simulink model "Torque_controller_IFOC"  (R2023b)
settings: Solver=ode5  StartTime=0.0  StopTime=tsim  FixedStep=tstep  MaxStep=1e-4  RelTol=1e-3
undefined symbols (not defined in the file or in its folder): MI_Contr, MI_contr, MI_motor, tau_L, tau_Rref
libraries: simulink x6, mcbcontrolslib x2, spsRMSLib x2
settings Model: Creator=HP  LastModifiedBy=HP

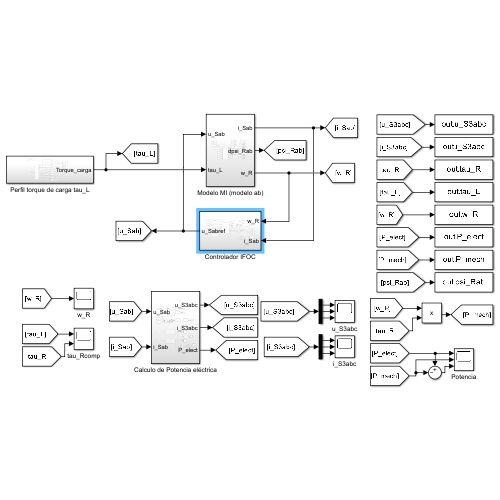
[thumbnail: Simulink's stored preview of the top-level diagram]
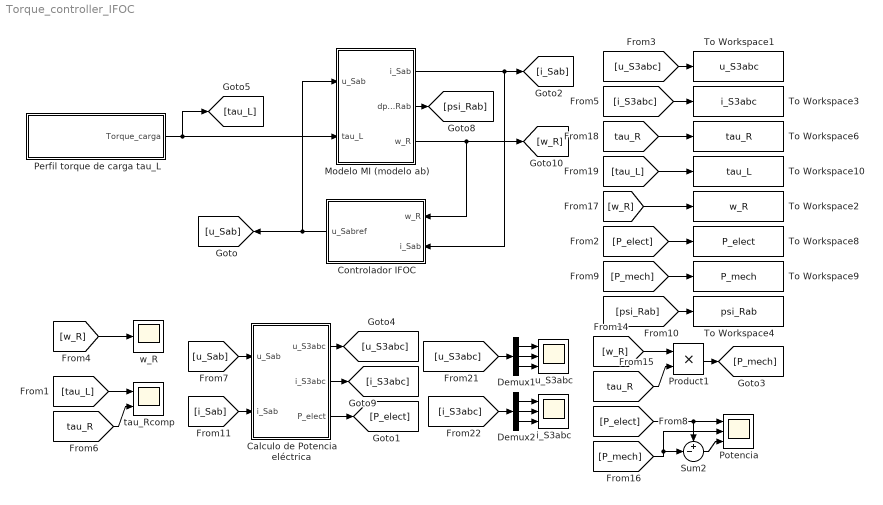
== system Torque_controller_IFOC ==
  Calculo de Potencia eléctrica : Subsystem
  Controlador IFOC : Subsystem
  Demux1 : Demux  Outputs=3
  Demux2 : Demux  Outputs=3
  Modelo MI (modelo ab) : Subsystem
  Perfil torque de carga tau_L : Subsystem
  Potencia : Scope  NumInputPorts=3
  Product1 : Product
  Sum2 : Sum  Inputs=+-|
  To Workspace1 : ToWorkspace  VariableName=u_S3abc  SaveFormat=Timeseries  SampleTime=-1
  To Workspace10 : ToWorkspace  VariableName=tau_L  SaveFormat=Timeseries  SampleTime=-1
  To Workspace2 : ToWorkspace  VariableName=w_R  SaveFormat=Timeseries  SampleTime=-1
  To Workspace3 : ToWorkspace  VariableName=i_S3abc  SaveFormat=Timeseries  SampleTime=-1
  To Workspace4 : ToWorkspace  VariableName=psi_Rab  SaveFormat=Timeseries  SampleTime=-1
  To Workspace6 : ToWorkspace  VariableName=tau_R  SaveFormat=Timeseries  SampleTime=-1
  To Workspace8 : ToWorkspace  VariableName=P_elect  SaveFormat=Timeseries  SampleTime=-1
  To Workspace9 : ToWorkspace  VariableName=P_mech  SaveFormat=Timeseries  SampleTime=-1
  i_S3abc : Scope  NumInputPorts=3
  tau_Rcomp : Scope  NumInputPorts=2
  u_S3abc : Scope  NumInputPorts=3
  w_R : Scope
  wires:
  Modelo MI (modelo ab)/1(i_Sab) -> [i_Sab], Controlador IFOC/2(i_Sab)
  Modelo MI (modelo ab)/3(w_R) -> Controlador IFOC/1(w_R), [w_R]
  Controlador IFOC/1(u_Sabref) -> Modelo MI (modelo ab)/1(u_Sab), [u_Sab]
  Modelo MI (modelo ab)/2(dpsi_Rab) -> [psi_Rab]
  Perfil torque de carga tau_L/1(Torque_carga) -> Modelo MI (modelo ab)/2(tau_L), [tau_L]
  Calculo de Potencia eléctrica/1(u_S3abc) -> [u_S3abc]
  Calculo de Potencia eléctrica/3(P_elect) -> [P_elect]
  Product1/1 -> [P_mech]
  [i_S3abc] -> Demux2/1
  [w_R] -> Product1/1
  [tau_R] -> Product1/2
  [P_elect] -> Potencia/1, Sum2/1
  [u_S3abc] -> Demux1/1
  Demux1/1 -> u_S3abc/1
  [i_Sab] -> Calculo de Potencia eléctrica/2(i_Sab)
  Calculo de Potencia eléctrica/2(i_S3abc) -> [i_S3abc]
  Sum2/1 -> Potencia/3
  Demux1/3 -> u_S3abc/3
  [P_mech] -> Potencia/2, Sum2/2
  Demux2/1 -> i_S3abc/1
  [tau_L] -> tau_Rcomp/1
  [tau_R] -> tau_Rcomp/2
  Demux2/2 -> i_S3abc/2
  Demux2/3 -> i_S3abc/3
  Demux1/2 -> u_S3abc/2
  [u_Sab] -> Calculo de Potencia eléctrica/1(u_Sab)
  [P_elect] -> To Workspace8/1
  [w_R] -> To Workspace2/1
  [i_S3abc] -> To Workspace3/1
  [psi_Rab] -> To Workspace4/1
  [tau_L] -> To Workspace10/1
  [P_mech] -> To Workspace9/1
  [tau_R] -> To Workspace6/1
  [u_S3abc] -> To Workspace1/1
  [w_R] -> w_R/1

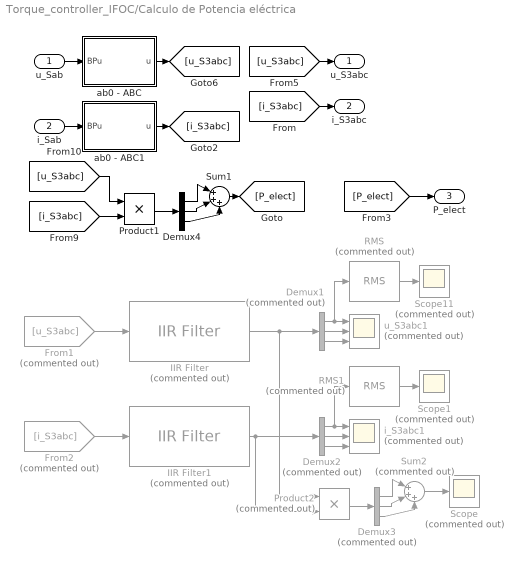
== system Torque_controller_IFOC/Calculo de Potencia eléctrica ==
  u_Sab : Inport
  i_Sab : Inport  Port=2
  Demux1 : Demux  Commented=on  Outputs=3
  Demux2 : Demux  Commented=on  Outputs=3
  Demux3 : Demux  Commented=on  Outputs=3
  Demux4 : Demux  Outputs=3
  From1 : From  Commented=on  GotoTag=u_S3abc
  From2 : From  Commented=on  GotoTag=i_S3abc
  IIR Filter : mcbcontrolslib/IIR Filter  Commented=on  VariantControl=Low Pass Filter  VariantSelect=Low-pass  Filter_constant=0.04  advancedSettings=on  Ts=50e-6  cutOff_freq=132.6291
      settings: LibrarySourceBlock=mcbhdllib/Signal Management/IIR Filter
  IIR Filter1 : mcbcontrolslib/IIR Filter  Commented=on  VariantControl=Low Pass Filter  VariantSelect=Low-pass  Filter_constant=0.04  advancedSettings=on  Ts=50e-6  cutOff_freq=132.6291
      settings: LibrarySourceBlock=mcbhdllib/Signal Management/IIR Filter
  Product1 : Product
  Product2 : Product  Commented=on
  RMS : spsRMSLib/RMS  Commented=on  TrueRMS=on  Freq=60  RMSInit=120  Ts=0
  RMS1 : spsRMSLib/RMS  Commented=on  TrueRMS=on  Freq=60  RMSInit=120  Ts=0
  Scope : Scope  Commented=on
  Scope1 : Scope  Commented=on
  Scope11 : Scope  Commented=on
  Sum1 : Sum  Inputs=|+++
  Sum2 : Sum  Commented=on  Inputs=|+++
  ab0 - ABC : MATLAB Function  TreatAsAtomicUnit=on
  ab0 - ABC1 : MATLAB Function  TreatAsAtomicUnit=on
  i_S3abc1 : Scope  Commented=on  NumInputPorts=3
  u_S3abc1 : Scope  Commented=on  NumInputPorts=3
  u_S3abc : Outport
  i_S3abc : Outport  Port=2
  P_elect : Outport  Port=3
  wires:
  Demux4/1 -> Sum1/1
  [i_S3abc] -> Product1/2
  i_Sab/1 -> ab0 - ABC1/1(BPu)
  Demux4/3 -> Sum1/3
  [u_S3abc] -> Product1/1
  Demux4/2 -> Sum1/2
  Product1/1 -> Demux4/1
  u_Sab/1 -> ab0 - ABC/1(BPu)
  [u_S3abc] -> u_S3abc/1
  [i_S3abc] -> i_S3abc/1
  ab0 - ABC/1(u) -> [u_S3abc]
  ab0 - ABC1/1(u) -> [i_S3abc]
  IIR Filter/1 -> Product2/1, Demux1/1
  RMS/1 -> Scope11/1
  Demux1/2 -> u_S3abc1/2
  Demux1/3 -> u_S3abc1/3
  Demux1/1 -> RMS/1, u_S3abc1/1
  From1/1 -> IIR Filter/1
  Demux2/1 -> RMS1/1, i_S3abc1/1
  RMS1/1 -> Scope1/1
  Demux2/2 -> i_S3abc1/2
  IIR Filter1/1 -> Product2/2, Demux2/1
  From2/1 -> IIR Filter1/1
  Demux2/3 -> i_S3abc1/3
  Demux3/2 -> Sum2/2
  Demux3/3 -> Sum2/3
  Sum2/1 -> Scope/1
  Product2/1 -> Demux3/1
  Demux3/1 -> Sum2/1
  Sum1/1 -> [P_elect]
  [P_elect] -> P_elect/1

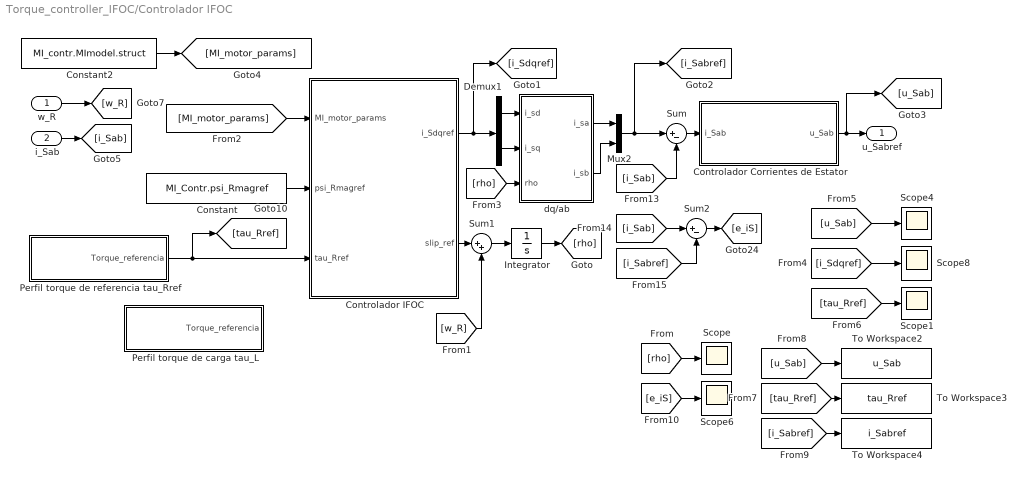
== system Torque_controller_IFOC/Controlador IFOC ==
  w_R : Inport
  i_Sab : Inport  Port=2
  Constant : Constant  Value=MI_Contr.psi_Rmagref
  Constant2 : Constant  Value=MI_contr.MImodel.struct  OutDataTypeStr=Bus: MI_bus
  Controlador Corrientes de Estator : Subsystem
  Controlador IFOC : MATLAB Function  TreatAsAtomicUnit=on
  Demux1 : Demux  Outputs=2
  Integrator : Integrator
  Mux2 : Mux  Inputs=2
  Perfil torque de carga tau_L : Subsystem
  Perfil torque de referencia tau_Rref : Subsystem
  Scope{,1,4,6,8} (5 alike) : Scope
  Sum : Sum  Inputs=|+-
  Sum1 : Sum  Inputs=|++
  Sum2 : Sum  Inputs=|+-
  To Workspace2 : ToWorkspace  VariableName=u_Sab  SaveFormat=Timeseries  SampleTime=-1
  To Workspace3 : ToWorkspace  VariableName=tau_Rref  SaveFormat=Timeseries  SampleTime=-1
  To Workspace4 : ToWorkspace  VariableName=i_Sabref  SaveFormat=Timeseries  SampleTime=-1
  dq/ab : MATLAB Function  TreatAsAtomicUnit=on
  u_Sabref : Outport
  wires:
  Controlador Corrientes de Estator/1(u_Sab) -> [u_Sab], u_Sabref/1
  [i_Sab] -> Sum/2
  Sum/1 -> Controlador Corrientes de Estator/1(i_Sab)
  dq/ab/2(i_sb) -> Mux2/2
  dq/ab/1(i_sa) -> Mux2/1
  Demux1/1 -> dq/ab/1(i_sd)
  Demux1/2 -> dq/ab/2(i_sq)
  Controlador IFOC/1(i_Sdqref) -> [i_Sdqref], Demux1/1
  i_Sab/1 -> [i_Sab]
  Controlador IFOC/2(slip_ref) -> Sum1/1
  w_R/1 -> [w_R]
  [w_R] -> Sum1/2
  Sum1/1 -> Integrator/1
  Integrator/1 -> [rho]
  [MI_motor_params] -> Controlador IFOC/1(MI_motor_params)
  Constant/1 -> Controlador IFOC/2(psi_Rmagref)
  [rho] -> dq/ab/3(rho)
  [i_Sdqref] -> Scope8/1
  [rho] -> Scope/1
  [u_Sab] -> Scope4/1
  [i_Sab] -> Sum2/1
  [i_Sabref] -> Sum2/2
  Mux2/1 -> [i_Sabref], Sum/1
  [tau_Rref] -> Scope1/1
  Perfil torque de referencia tau_Rref/1(Torque_referencia) -> Controlador IFOC/3(tau_Rref), [tau_Rref]
  [u_Sab] -> To Workspace2/1
  [tau_Rref] -> To Workspace3/1
  [i_Sabref] -> To Workspace4/1
  Sum2/1 -> [e_iS]
  [e_iS] -> Scope6/1
  Constant2/1 -> [MI_motor_params]

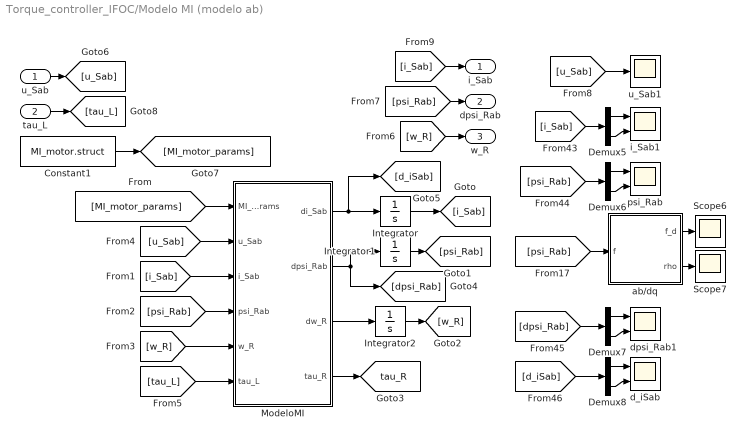
== system Torque_controller_IFOC/Modelo MI (modelo ab) ==
  u_Sab : Inport
  tau_L : Inport  Port=2
  Constant1 : Constant  Value=MI_motor.struct  OutDataTypeStr=Bus: MI_bus
  Demux{5..8} (4 alike) : Demux  Outputs=2
  Integrator : Integrator
  Integrator1 : Integrator
  Integrator2 : Integrator
  ModeloMI : MATLAB Function  TreatAsAtomicUnit=on
  Scope6 : Scope
  Scope7 : Scope
  ab/dq : MATLAB Function  TreatAsAtomicUnit=on
  d_iSab : Scope  NumInputPorts=2
  dpsi_Rab1 : Scope  NumInputPorts=2
  i_Sab1 : Scope  NumInputPorts=2
  psi_Rab : Scope  NumInputPorts=2
  u_Sab1 : Scope
  i_Sab : Outport
  dpsi_Rab : Outport  Port=2
  w_R : Outport  Port=3
  tag scope: tau_R=global
  wires:
  ModeloMI/1(di_Sab) -> Integrator/1, [d_iSab]
  ModeloMI/2(dpsi_Rab) -> [dpsi_Rab], Integrator1/1
  [w_R] -> ModeloMI/5(w_R)
  [psi_Rab] -> ModeloMI/4(psi_Rab)
  Integrator2/1 -> [w_R]
  [i_Sab] -> ModeloMI/3(i_Sab)
  ModeloMI/3(dw_R) -> Integrator2/1
  Integrator1/1 -> [psi_Rab]
  u_Sab/1 -> [u_Sab]
  ModeloMI/4(tau_R) -> [tau_R]
  Demux7/1 -> dpsi_Rab1/1
  Demux7/2 -> dpsi_Rab1/2
  [d_iSab] -> Demux8/1
  Demux8/2 -> d_iSab/2
  Demux8/1 -> d_iSab/1
  [dpsi_Rab] -> Demux7/1
  Integrator/1 -> [i_Sab]
  [MI_motor_params] -> ModeloMI/1(MI_motor_params)
  Constant1/1 -> [MI_motor_params]
  Demux6/2 -> psi_Rab/2
  Demux5/1 -> i_Sab1/1
  [psi_Rab] -> Demux6/1
  Demux5/2 -> i_Sab1/2
  Demux6/1 -> psi_Rab/1
  [u_Sab] -> u_Sab1/1
  [i_Sab] -> Demux5/1
  ab/dq/2(rho) -> Scope7/1
  ab/dq/1(f_d) -> Scope6/1
  [psi_Rab] -> ab/dq/1(f)
  [u_Sab] -> ModeloMI/2(u_Sab)
  tau_L/1 -> [tau_L]
  [tau_L] -> ModeloMI/6(tau_L)
  [i_Sab] -> i_Sab/1
  [psi_Rab] -> dpsi_Rab/1
  [w_R] -> w_R/1

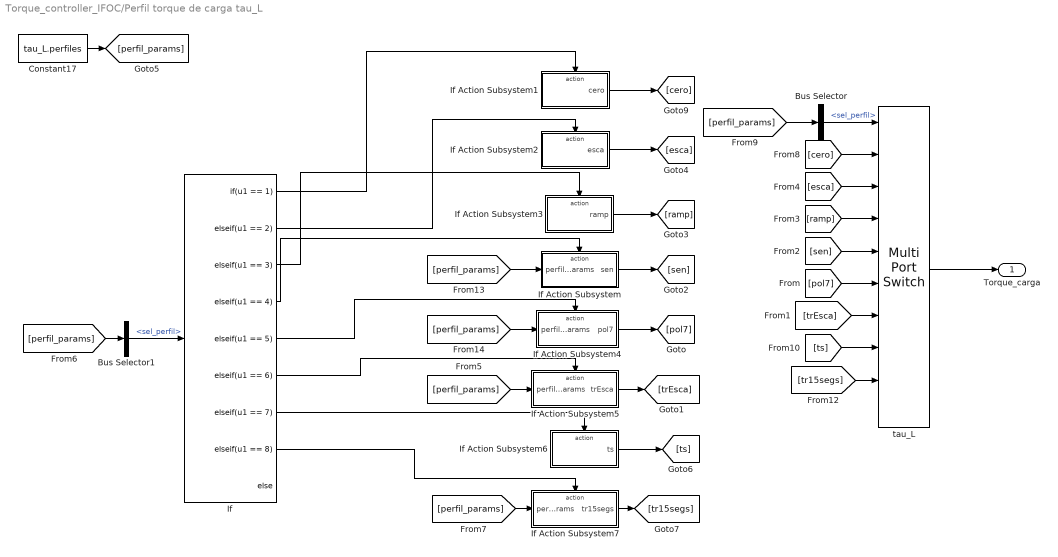
== system Torque_controller_IFOC/Perfil torque de carga tau_L ==
  Bus Selector : BusSelector  OutputSignals=sel_perfil
  Bus Selector1 : BusSelector  OutputSignals=sel_perfil
  Constant17 : Constant  Value=tau_L.perfiles  OutDataTypeStr=Bus: Perfil_bus
  If : If  IfExpression=u1 == 1  ElseIfExpressions=u1 == 2,u1 == 3,u1 == 4,u1 == 5,u1 == 6,u1 == 7,u1 == 8
  If Action Subsystem : Subsystem  TreatAsAtomicUnit=on
  If Action Subsystem1 : Subsystem  TreatAsAtomicUnit=on
  If Action Subsystem2 : Subsystem  TreatAsAtomicUnit=on
  If Action Subsystem3 : Subsystem  TreatAsAtomicUnit=on
  If Action Subsystem4 : Subsystem  TreatAsAtomicUnit=on
  If Action Subsystem5 : Subsystem  TreatAsAtomicUnit=on
  If Action Subsystem6 : Subsystem  TreatAsAtomicUnit=on
  If Action Subsystem7 : Subsystem  TreatAsAtomicUnit=on
  tau_L : MultiPortSwitch  Inputs=9  SaturateOnIntegerOverflow=off  InputSameDT=off
  Torque_carga : Outport
  wires:
  tau_L/1 -> Torque_carga/1
  [ramp] -> tau_L/4
  [trEsca] -> tau_L/7
  [pol7] -> tau_L/6
  [sen] -> tau_L/5
  [esca] -> tau_L/3
  Constant17/1 -> [perfil_params]
  [ts] -> tau_L/8
  [tr15segs] -> tau_L/9
  Bus Selector/1 -> tau_L/1  "<sel_perfil>"
  [perfil_params] -> Bus Selector/1
  If Action Subsystem/1(sen) -> [sen]
  [perfil_params] -> Bus Selector1/1
  Bus Selector1/1 -> If/1  "<sel_perfil>"
  If/4 -> If Action Subsystem/Action
  If Action Subsystem1/1(cero) -> [cero]
  [cero] -> tau_L/2
  [perfil_params] -> If Action Subsystem/1(perfil_params)
  If/1 -> If Action Subsystem1/Action
  If Action Subsystem2/1(esca) -> [esca]
  If/2 -> If Action Subsystem2/Action
  If Action Subsystem3/1(ramp) -> [ramp]
  If/3 -> If Action Subsystem3/Action
  [perfil_params] -> If Action Subsystem4/1(perfil_params)
  If/5 -> If Action Subsystem4/Action
  If Action Subsystem4/1(pol7) -> [pol7]
  If Action Subsystem5/1(trEsca) -> [trEsca]
  [perfil_params] -> If Action Subsystem5/1(perfil_params)
  If Action Subsystem6/1(ts) -> [ts]
  If/6 -> If Action Subsystem5/Action
  If/7 -> If Action Subsystem6/Action
  If Action Subsystem7/1(tr15segs) -> [tr15segs]
  If/8 -> If Action Subsystem7/Action
  [perfil_params] -> If Action Subsystem7/1(perfil_params)

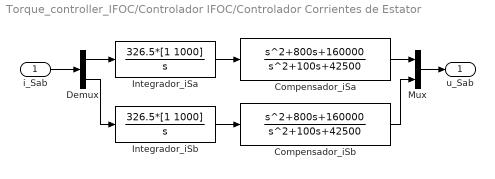
== system Torque_controller_IFOC/Controlador IFOC/Controlador Corrientes de Estator ==
  i_Sab : Inport
  Compensador_iSa : TransferFcn  Numerator=[1,800,160000]  Denominator=[1,100,42500]
  Compensador_iSb : TransferFcn  Numerator=[1,800,160000]  Denominator=[1,100,42500]
  Demux : Demux  Outputs=2
  Integrador_iSa : TransferFcn  Numerator=326.5*[1 1000]  Denominator=[1 0]
  Integrador_iSb : TransferFcn  Numerator=326.5*[1 1000]  Denominator=[1 0]
  Mux : Mux  Inputs=2
  u_Sab : Outport
  wires:
  Integrador_iSa/1 -> Compensador_iSa/1
  Integrador_iSb/1 -> Compensador_iSb/1
  i_Sab/1 -> Demux/1
  Demux/1 -> Integrador_iSa/1
  Demux/2 -> Integrador_iSb/1
  Compensador_iSa/1 -> Mux/1
  Mux/1 -> u_Sab/1
  Compensador_iSb/1 -> Mux/2

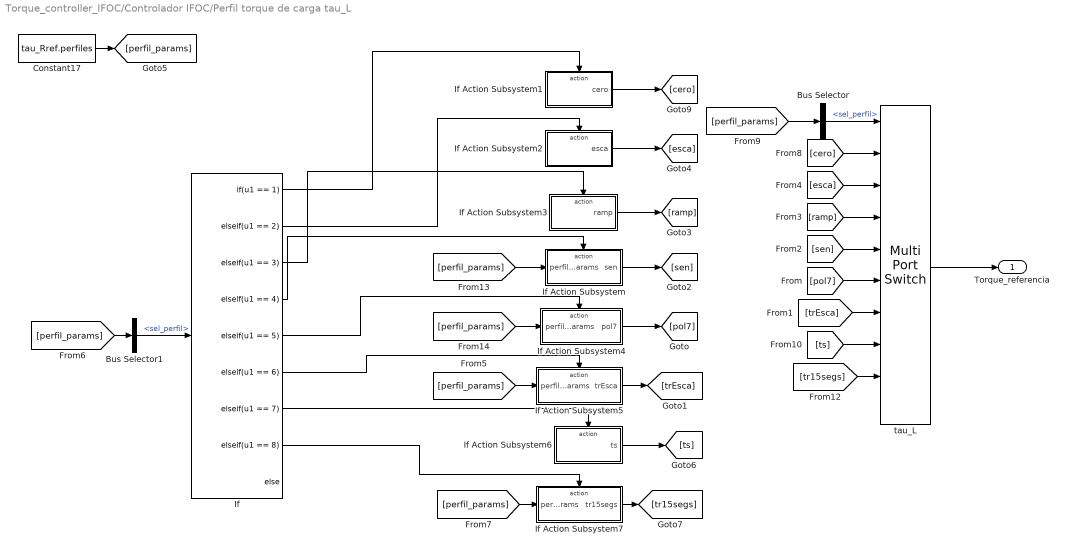
== system Torque_controller_IFOC/Controlador IFOC/Perfil torque de carga tau_L ==
  Bus Selector : BusSelector  OutputSignals=sel_perfil
  Bus Selector1 : BusSelector  OutputSignals=sel_perfil
  Constant17 : Constant  Value=tau_Rref.perfiles  OutDataTypeStr=Bus: Perfil_bus
  If : If  IfExpression=u1 == 1  ElseIfExpressions=u1 == 2,u1 == 3,u1 == 4,u1 == 5,u1 == 6,u1 == 7,u1 == 8
  If Action Subsystem : Subsystem  TreatAsAtomicUnit=on
  If Action Subsystem1 : Subsystem  TreatAsAtomicUnit=on
  If Action Subsystem2 : Subsystem  TreatAsAtomicUnit=on
  If Action Subsystem3 : Subsystem  TreatAsAtomicUnit=on
  If Action Subsystem4 : Subsystem  TreatAsAtomicUnit=on
  If Action Subsystem5 : Subsystem  TreatAsAtomicUnit=on
  If Action Subsystem6 : Subsystem  TreatAsAtomicUnit=on
  If Action Subsystem7 : Subsystem  TreatAsAtomicUnit=on
  tau_L : MultiPortSwitch  Inputs=9  SaturateOnIntegerOverflow=off  InputSameDT=off
  Torque_referencia : Outport
  wires:
  tau_L/1 -> Torque_referencia/1
  [ramp] -> tau_L/4
  [trEsca] -> tau_L/7
  [pol7] -> tau_L/6
  [sen] -> tau_L/5
  [esca] -> tau_L/3
  Constant17/1 -> [perfil_params]
  [ts] -> tau_L/8
  [tr15segs] -> tau_L/9
  Bus Selector/1 -> tau_L/1  "<sel_perfil>"
  [perfil_params] -> Bus Selector/1
  If Action Subsystem/1(sen) -> [sen]
  [perfil_params] -> Bus Selector1/1
  Bus Selector1/1 -> If/1  "<sel_perfil>"
  If/4 -> If Action Subsystem/Action
  If Action Subsystem1/1(cero) -> [cero]
  [cero] -> tau_L/2
  [perfil_params] -> If Action Subsystem/1(perfil_params)
  If/1 -> If Action Subsystem1/Action
  If Action Subsystem2/1(esca) -> [esca]
  If/2 -> If Action Subsystem2/Action
  If Action Subsystem3/1(ramp) -> [ramp]
  If/3 -> If Action Subsystem3/Action
  [perfil_params] -> If Action Subsystem4/1(perfil_params)
  If/5 -> If Action Subsystem4/Action
  If Action Subsystem4/1(pol7) -> [pol7]
  If Action Subsystem5/1(trEsca) -> [trEsca]
  [perfil_params] -> If Action Subsystem5/1(perfil_params)
  If Action Subsystem6/1(ts) -> [ts]
  If/6 -> If Action Subsystem5/Action
  If/7 -> If Action Subsystem6/Action
  If Action Subsystem7/1(tr15segs) -> [tr15segs]
  If/8 -> If Action Subsystem7/Action
  [perfil_params] -> If Action Subsystem7/1(perfil_params)

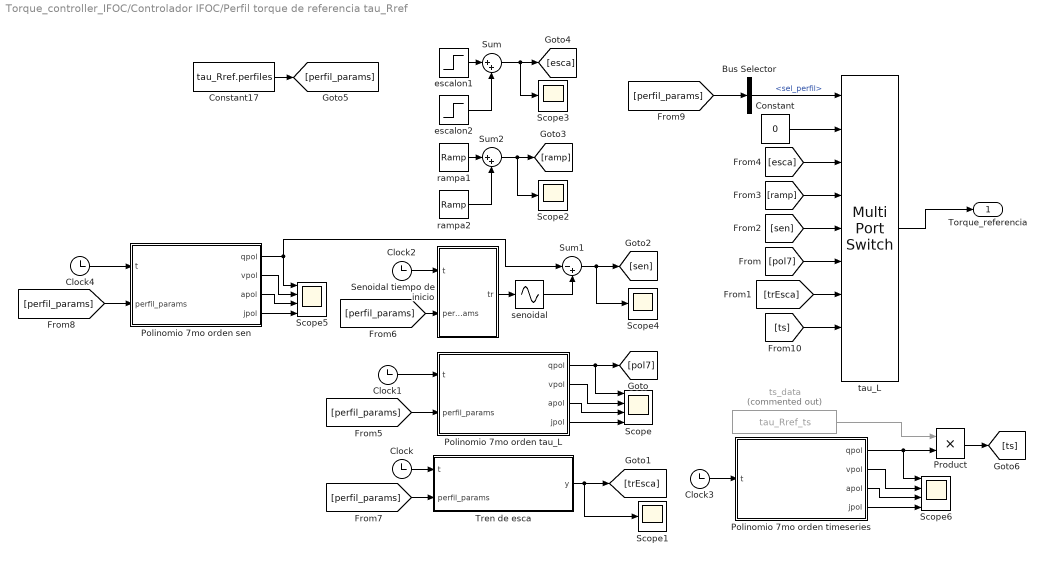
== system Torque_controller_IFOC/Controlador IFOC/Perfil torque de referencia tau_Rref ==
  Bus Selector : BusSelector  OutputSignals=sel_perfil
  Clock{,1..4} (5 alike) : Clock
  Constant : Constant  Value=0
  Constant17 : Constant  Value=tau_Rref.perfiles  OutDataTypeStr=Bus: Perfil_bus
  Polinomio 7mo orden sen : MATLAB Function  TreatAsAtomicUnit=on
  Polinomio 7mo orden tau_L : MATLAB Function  TreatAsAtomicUnit=on
  Polinomio 7mo orden timeseries : MATLAB Function  TreatAsAtomicUnit=on
  Product : Product
  Scope : Scope  NumInputPorts=4
  Scope{1..4} (4 alike) : Scope
  Scope5 : Scope  NumInputPorts=4
  Scope6 : Scope  NumInputPorts=4
  Senoidal tiempo de inicio : MATLAB Function  TreatAsAtomicUnit=on
  Sum : Sum  Inputs=|++
  Sum1 : Sum  Inputs=|-+
  Sum2 : Sum  Inputs=|++
  Tren de esca : MATLAB Function  TreatAsAtomicUnit=on
  escalon1 : Step  Time=2.5  After=0.85  SampleTime=0
  escalon2 : Step  Time=7.5  After=-0.85  SampleTime=0
  rampa1 : simulink/Sources/Ramp  slope=0.02064  start=2.5  InitialOutput=0
  rampa2 : simulink/Sources/Ramp  slope=-0.02064  start=7.5  InitialOutput=0
  senoidal : Sin  TimeSource=Use external signal  Amplitude=0.41519  Frequency=6.2832  Phase=1.5708  SampleTime=0
  tau_L : MultiPortSwitch  Inputs=8  SaturateOnIntegerOverflow=off  InputSameDT=off
  ts_data : FromWorkspace  Commented=on  VariableName=tau_Rref_ts
  Torque_referencia : Outport
  wires:
  Polinomio 7mo orden tau_L/2(vpol) -> Scope/2
  Polinomio 7mo orden tau_L/3(apol) -> Scope/3
  Polinomio 7mo orden tau_L/4(jpol) -> Scope/4
  Sum2/1 -> Scope2/1, [ramp]
  Constant/1 -> tau_L/2
  rampa2/1 -> Sum2/2
  rampa1/1 -> Sum2/1
  tau_L/1 -> Torque_referencia/1
  Clock/1 -> Tren de esca/1(t)
  Tren de esca/1(y) -> Scope1/1, [trEsca]
  Polinomio 7mo orden tau_L/1(qpol) -> Scope/1, [pol7]
  escalon1/1 -> Sum/1
  Sum/1 -> [esca], Scope3/1
  escalon2/1 -> Sum/2
  [ramp] -> tau_L/4
  [trEsca] -> tau_L/7
  [pol7] -> tau_L/6
  [sen] -> tau_L/5
  [esca] -> tau_L/3
  Clock2/1 -> Senoidal tiempo de inicio/1(t)
  Senoidal tiempo de inicio/1(tr) -> senoidal/1
  Constant17/1 -> [perfil_params]
  Clock1/1 -> Polinomio 7mo orden tau_L/1(t)
  [perfil_params] -> Polinomio 7mo orden tau_L/2(perfil_params)
  [perfil_params] -> Senoidal tiempo de inicio/2(perfil_params)
  [perfil_params] -> Tren de esca/2(perfil_params)
  Clock4/1 -> Polinomio 7mo orden sen/1(t)
  [perfil_params] -> Polinomio 7mo orden sen/2(perfil_params)
  senoidal/1 -> Sum1/2
  Polinomio 7mo orden sen/2(vpol) -> Scope5/2
  Polinomio 7mo orden sen/3(apol) -> Scope5/3
  Polinomio 7mo orden sen/4(jpol) -> Scope5/4
  Polinomio 7mo orden sen/1(qpol) -> Sum1/1, Scope5/1
  Sum1/1 -> Scope4/1, [sen]
  Bus Selector/1 -> tau_L/1  "<sel_perfil>"
  [perfil_params] -> Bus Selector/1
  Clock3/1 -> Polinomio 7mo orden timeseries/1(t)
  Polinomio 7mo orden timeseries/2(vpol) -> Scope6/2
  Polinomio 7mo orden timeseries/1(qpol) -> Product/2, Scope6/1
  Polinomio 7mo orden timeseries/4(jpol) -> Scope6/4
  Polinomio 7mo orden timeseries/3(apol) -> Scope6/3
  ts_data/1 -> Product/1
  Product/1 -> [ts]
  [ts] -> tau_L/8

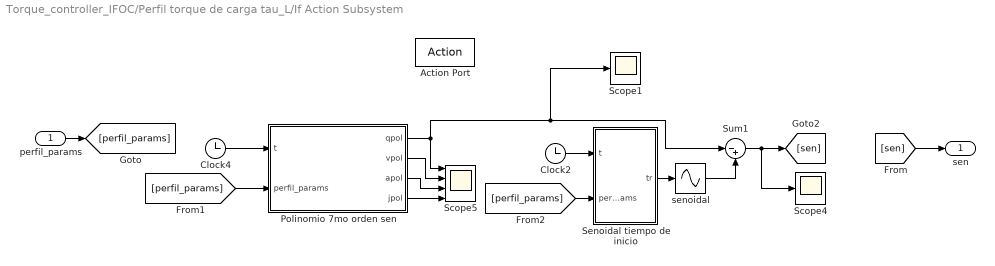
== system Torque_controller_IFOC/Perfil torque de carga tau_L/If Action Subsystem ==
  perfil_params : Inport
  Action Port : ActionPort
  Clock2 : Clock
  Clock4 : Clock
  Polinomio 7mo orden sen : MATLAB Function  TreatAsAtomicUnit=on
  Scope1 : Scope
  Scope4 : Scope
  Scope5 : Scope  NumInputPorts=4
  Senoidal tiempo de inicio : MATLAB Function  TreatAsAtomicUnit=on
  Sum1 : Sum  Inputs=|-+
  senoidal : Sin  TimeSource=Use external signal  Frequency=6.2832  Phase=1.5708  SampleTime=0
  sen : Outport
  wires:
  Clock4/1 -> Polinomio 7mo orden sen/1(t)
  Polinomio 7mo orden sen/1(qpol) -> Scope1/1, Sum1/1, Scope5/1
  Sum1/1 -> Scope4/1, [sen]
  Polinomio 7mo orden sen/4(jpol) -> Scope5/4
  Polinomio 7mo orden sen/3(apol) -> Scope5/3
  Clock2/1 -> Senoidal tiempo de inicio/1(t)
  [perfil_params] -> Polinomio 7mo orden sen/2(perfil_params)
  Polinomio 7mo orden sen/2(vpol) -> Scope5/2
  senoidal/1 -> Sum1/2
  Senoidal tiempo de inicio/1(tr) -> senoidal/1
  [sen] -> sen/1
  perfil_params/1 -> [perfil_params]
  [perfil_params] -> Senoidal tiempo de inicio/2(perfil_params)

== system Torque_controller_IFOC/Perfil torque de carga tau_L/If Action Subsystem1 ==
  Action Port : ActionPort
  Constant : Constant  Value=0
  cero : Outport
  wires:
  Constant/1 -> cero/1

== system Torque_controller_IFOC/Perfil torque de carga tau_L/If Action Subsystem2 ==
  Action Port : ActionPort
  Scope3 : Scope
  Sum : Sum  Inputs=|++
  escalon1 : Step  Time=2.5  After=0.70582  SampleTime=0
  escalon2 : Step  Time=7.5  After=-0.70582  SampleTime=0
  esca : Outport
  wires:
  escalon2/1 -> Sum/2
  escalon1/1 -> Sum/1
  Sum/1 -> [esca], Scope3/1
  [esca] -> esca/1

== system Torque_controller_IFOC/Perfil torque de carga tau_L/If Action Subsystem3 ==
  Action Port : ActionPort
  Scope2 : Scope
  Sum2 : Sum  Inputs=|++
  rampa1 : simulink/Sources/Ramp  slope=0.02064  start=2.5  InitialOutput=0
  rampa2 : simulink/Sources/Ramp  slope=-0.02064  start=7.5  InitialOutput=0
  ramp : Outport
  wires:
  rampa2/1 -> Sum2/2
  rampa1/1 -> Sum2/1
  Sum2/1 -> Scope2/1, [ramp]
  [ramp] -> ramp/1

== system Torque_controller_IFOC/Perfil torque de carga tau_L/If Action Subsystem4 ==
  perfil_params : Inport
  Action Port : ActionPort
  Clock1 : Clock
  Polinomio 7mo orden tau_L : MATLAB Function  TreatAsAtomicUnit=on
  Scope : Scope  NumInputPorts=4
  pol7 : Outport
  wires:
  Polinomio 7mo orden tau_L/4(jpol) -> Scope/4
  Polinomio 7mo orden tau_L/1(qpol) -> Scope/1, [pol7]
  Polinomio 7mo orden tau_L/2(vpol) -> Scope/2
  Clock1/1 -> Polinomio 7mo orden tau_L/1(t)
  Polinomio 7mo orden tau_L/3(apol) -> Scope/3
  perfil_params/1 -> Polinomio 7mo orden tau_L/2(perfil_params)
  [pol7] -> pol7/1

== system Torque_controller_IFOC/Perfil torque de carga tau_L/If Action Subsystem5 ==
  perfil_params : Inport
  Action Port : ActionPort
  Clock : Clock
  Scope1 : Scope
  Tren de esca : MATLAB Function  TreatAsAtomicUnit=on
  trEsca : Outport
  wires:
  Tren de esca/1(q) -> Scope1/1, [trEsca]
  Clock/1 -> Tren de esca/1(t)
  perfil_params/1 -> Tren de esca/2(perfil_params)
  [trEsca] -> trEsca/1

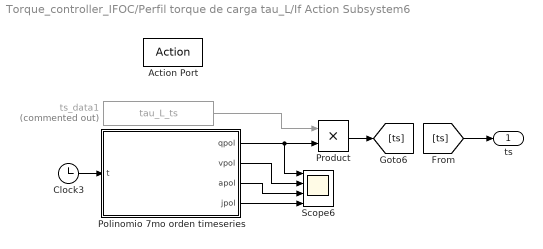
== system Torque_controller_IFOC/Perfil torque de carga tau_L/If Action Subsystem6 ==
  Action Port : ActionPort
  Clock3 : Clock
  Polinomio 7mo orden timeseries : MATLAB Function  TreatAsAtomicUnit=on
  Product : Product
  Scope6 : Scope  NumInputPorts=4
  ts_data1 : FromWorkspace  Commented=on  VariableName=tau_L_ts
  ts : Outport
  wires:
  Product/1 -> [ts]
  Clock3/1 -> Polinomio 7mo orden timeseries/1(t)
  ts_data1/1 -> Product/1
  Polinomio 7mo orden timeseries/4(jpol) -> Scope6/4
  Polinomio 7mo orden timeseries/2(vpol) -> Scope6/2
  Polinomio 7mo orden timeseries/3(apol) -> Scope6/3
  Polinomio 7mo orden timeseries/1(qpol) -> Product/2, Scope6/1
  [ts] -> ts/1

== system Torque_controller_IFOC/Perfil torque de carga tau_L/If Action Subsystem7 ==
  perfil_params : Inport
  Action Port : ActionPort
  Clock5 : Clock
  Scope7 : Scope
  Trayectoria 15 segmentos : MATLAB Function  TreatAsAtomicUnit=on
  tr15segs : Outport
  wires:
  Clock5/1 -> Trayectoria 15 segmentos/1(t)
  Trayectoria 15 segmentos/1(q) -> Scope7/1, [tr15segs]
  [tr15segs] -> tr15segs/1
  perfil_params/1 -> Trayectoria 15 segmentos/2(perfil_params)

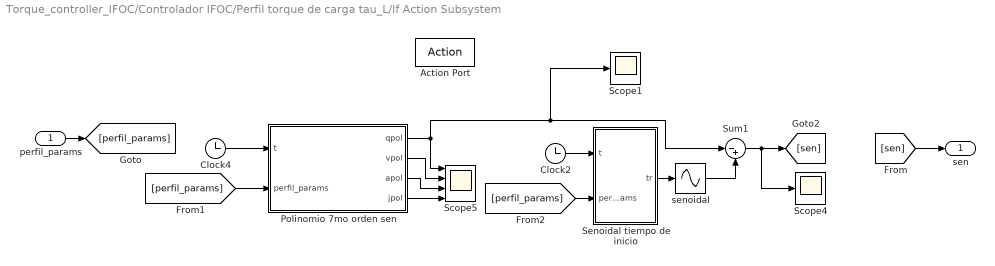
== system Torque_controller_IFOC/Controlador IFOC/Perfil torque de carga tau_L/If Action Subsystem ==
  perfil_params : Inport
  Action Port : ActionPort
  Clock2 : Clock
  Clock4 : Clock
  Polinomio 7mo orden sen : MATLAB Function  TreatAsAtomicUnit=on
  Scope1 : Scope
  Scope4 : Scope
  Scope5 : Scope  NumInputPorts=4
  Senoidal tiempo de inicio : MATLAB Function  TreatAsAtomicUnit=on
  Sum1 : Sum  Inputs=|-+
  senoidal : Sin  TimeSource=Use external signal  Frequency=6.2832  Phase=1.5708  SampleTime=0
  sen : Outport
  wires:
  Clock4/1 -> Polinomio 7mo orden sen/1(t)
  Polinomio 7mo orden sen/1(qpol) -> Scope1/1, Sum1/1, Scope5/1
  Sum1/1 -> Scope4/1, [sen]
  Polinomio 7mo orden sen/4(jpol) -> Scope5/4
  Polinomio 7mo orden sen/3(apol) -> Scope5/3
  Clock2/1 -> Senoidal tiempo de inicio/1(t)
  [perfil_params] -> Polinomio 7mo orden sen/2(perfil_params)
  Polinomio 7mo orden sen/2(vpol) -> Scope5/2
  senoidal/1 -> Sum1/2
  Senoidal tiempo de inicio/1(tr) -> senoidal/1
  [sen] -> sen/1
  perfil_params/1 -> [perfil_params]
  [perfil_params] -> Senoidal tiempo de inicio/2(perfil_params)

== system Torque_controller_IFOC/Controlador IFOC/Perfil torque de carga tau_L/If Action Subsystem1 ==
  Action Port : ActionPort
  Constant : Constant  Value=0
  cero : Outport
  wires:
  Constant/1 -> cero/1

== system Torque_controller_IFOC/Controlador IFOC/Perfil torque de carga tau_L/If Action Subsystem2 ==
  Action Port : ActionPort
  Scope3 : Scope
  Sum : Sum  Inputs=|++
  escalon1 : Step  Time=2.5  After=0.70582  SampleTime=0
  escalon2 : Step  Time=7.5  After=-0.70582  SampleTime=0
  esca : Outport
  wires:
  escalon2/1 -> Sum/2
  escalon1/1 -> Sum/1
  Sum/1 -> [esca], Scope3/1
  [esca] -> esca/1

== system Torque_controller_IFOC/Controlador IFOC/Perfil torque de carga tau_L/If Action Subsystem3 ==
  Action Port : ActionPort
  Scope2 : Scope
  Sum2 : Sum  Inputs=|++
  rampa1 : simulink/Sources/Ramp  slope=0.02064  start=2.5  InitialOutput=0
  rampa2 : simulink/Sources/Ramp  slope=-0.02064  start=7.5  InitialOutput=0
  ramp : Outport
  wires:
  rampa2/1 -> Sum2/2
  rampa1/1 -> Sum2/1
  Sum2/1 -> Scope2/1, [ramp]
  [ramp] -> ramp/1

== system Torque_controller_IFOC/Controlador IFOC/Perfil torque de carga tau_L/If Action Subsystem4 ==
  perfil_params : Inport
  Action Port : ActionPort
  Clock1 : Clock
  Polinomio 7mo orden tau_L : MATLAB Function  TreatAsAtomicUnit=on
  Scope : Scope  NumInputPorts=4
  pol7 : Outport
  wires:
  Polinomio 7mo orden tau_L/4(jpol) -> Scope/4
  Polinomio 7mo orden tau_L/1(qpol) -> Scope/1, [pol7]
  Polinomio 7mo orden tau_L/2(vpol) -> Scope/2
  Clock1/1 -> Polinomio 7mo orden tau_L/1(t)
  Polinomio 7mo orden tau_L/3(apol) -> Scope/3
  perfil_params/1 -> Polinomio 7mo orden tau_L/2(perfil_params)
  [pol7] -> pol7/1

== system Torque_controller_IFOC/Controlador IFOC/Perfil torque de carga tau_L/If Action Subsystem5 ==
  perfil_params : Inport
  Action Port : ActionPort
  Clock : Clock
  Scope1 : Scope
  Tren de esca : MATLAB Function  TreatAsAtomicUnit=on
  trEsca : Outport
  wires:
  Tren de esca/1(q) -> Scope1/1, [trEsca]
  Clock/1 -> Tren de esca/1(t)
  perfil_params/1 -> Tren de esca/2(perfil_params)
  [trEsca] -> trEsca/1

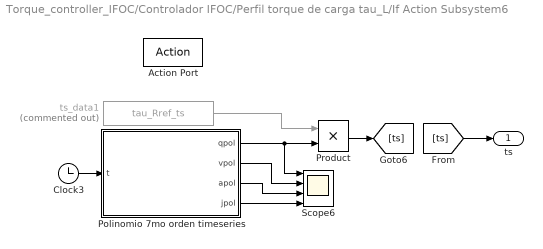
== system Torque_controller_IFOC/Controlador IFOC/Perfil torque de carga tau_L/If Action Subsystem6 ==
  Action Port : ActionPort
  Clock3 : Clock
  Polinomio 7mo orden timeseries : MATLAB Function  TreatAsAtomicUnit=on
  Product : Product
  Scope6 : Scope  NumInputPorts=4
  ts_data1 : FromWorkspace  Commented=on  VariableName=tau_Rref_ts
  ts : Outport
  wires:
  Product/1 -> [ts]
  Clock3/1 -> Polinomio 7mo orden timeseries/1(t)
  ts_data1/1 -> Product/1
  Polinomio 7mo orden timeseries/4(jpol) -> Scope6/4
  Polinomio 7mo orden timeseries/2(vpol) -> Scope6/2
  Polinomio 7mo orden timeseries/3(apol) -> Scope6/3
  Polinomio 7mo orden timeseries/1(qpol) -> Product/2, Scope6/1
  [ts] -> ts/1

== system Torque_controller_IFOC/Controlador IFOC/Perfil torque de carga tau_L/If Action Subsystem7 ==
  perfil_params : Inport
  Action Port : ActionPort
  Clock5 : Clock
  Scope7 : Scope
  Trayectoria 15 segmentos : MATLAB Function  TreatAsAtomicUnit=on
  tr15segs : Outport
  wires:
  Clock5/1 -> Trayectoria 15 segmentos/1(t)
  Trayectoria 15 segmentos/1(q) -> Scope7/1, [tr15segs]
  [tr15segs] -> tr15segs/1
  perfil_params/1 -> Trayectoria 15 segmentos/2(perfil_params)

== matlab function Torque_controller_IFOC/Controlador IFOC/Controlador IFOC ==
  data: MI_motor_params input; psi_Rmagref input; i_Sdqref output size=[2 1]; tau_Rref input; slip_ref output
function [i_Sdqref,slip_ref] = fcn(MI_motor_params,psi_Rmagref,tau_Rref)

[i_Sdqref,slip_ref] = IFOC_Torque_Controller.torque_controller(MI_motor_params,psi_Rmagref,tau_Rref);

== matlab function Torque_controller_IFOC/Controlador IFOC/Perfil torque de referencia tau_Rref/Polinomio 7mo orden sen ==
  data: t input; perfil_params input; qpol output; vpol output; apol output; jpol output
function [qpol,vpol,apol,jpol] = fcn(t,perfil_params)


% t,q0,q1,v0,v1,ac0,ac1,j0,j1,t0,t1)
%Trayectoria de referencia

q0 = 0;
q1 = perfil_params.senoidal.amplitud;

v0 = perfil_params.polinomio7.vel.inicial;
v1 = perfil_params.polinomio7.vel.final;

ac0 = perfil_params.polinomio7.acel.inicial;
ac1 = perfil_params.polinomio7.acel.final;

j0 = perfil_params.polinomio7.jerk.inicial;
j1 = perfil_params.polinomio7.jerk.inicial;

t0 = 0;
if perfil_params.senoidal.tiempo_inicio-1>0
    t0 = perfil_params.senoidal.tiempo_inicio-1;
else
    t0 = 0;
end

t1 = perfil_params.senoidal.tiempo_inicio;

% Coeficientes de un polinomio de 7mo grado

h = q1 - q0;
T = t1 - t0;

a = zeros(7+1,1);

a(1) = q0;
a(2) = v0;
a(3) = ac0/2;
a(4) = j0/6;
a(5) = (210*h-T*((30*ac0-15*ac1)*T+(4*j0+j1)*T^2+120*v0+90*v1))/(6*T^4);
a(6) = (-168*h-T*((20*ac0-14*ac1)*T+(2*j0+j1)*T^2+90*v0+78*v1))/(2*T^5);
a(7) = (420*h-T*((45*ac0-39*ac1)*T+(4*j0+3*j1)*T^2+216*v0+204*v1))/(6*T^6);
a(8) = (-120*h-T*((12*ac0-12*ac1)*T+(j0+j1)*T^2+60*v0+60*v1))/(6*T^7);

qa = flip(a')';
va = polyder(qa')';
aa = polyder(va')';
ja = polyder(aa')';


if t>=t0 && t<t1
    qpol = polyval(qa,t-t0);
    vpol = polyval(va,t-t0);
    apol = polyval(aa,t-t0);
    jpol = polyval(ja,t-t0);
elseif t>=t1
    qpol = polyval(qa,T);
    vpol = polyval(va,T);
    apol = polyval(aa,T);
    jpol = polyval(ja,T);
else
    qpol = 0;
    vpol = 0;
    apol = 0;
    jpol = 0;
end


qpol = perfil_params.senoidal.amplitud - qpol;

== matlab function Torque_controller_IFOC/Controlador IFOC/Perfil torque de referencia tau_Rref/Senoidal tiempo de inicio ==
  data: t input; tr output; perfil_params input
function tr = fcn(t,perfil_params)

t1 = perfil_params.senoidal.tiempo_inicio;

if t < t1
    tr = 0;
else
    tr = t - t1;
end

== matlab function Torque_controller_IFOC/Controlador IFOC/Perfil torque de referencia tau_Rref/Tren de esca ==
  data: t input; y output; perfil_params input
function y = fcn(t,perfil_params)

referencia = perfil_params.valor_referencia;
amplitud = perfil_params.escalones.amplitud;
tstep = perfil_params.escalones.tiempo_entre_escalones;


num_escalones = ceil(referencia/amplitud);

if floor(t/tstep)<num_escalones
    y = amplitud*floor(t/tstep);
else
    y = amplitud*num_escalones;
end

== matlab function Torque_controller_IFOC/Perfil torque de carga tau_L/If Action Subsystem/Polinomio 7mo orden sen ==
  data: t input; perfil_params input; qpol output; vpol output; apol output; jpol output
function [qpol,vpol,apol,jpol] = fcn(t,perfil_params)

%Trayectoria de referencia

q0 = 0;
q1 = perfil_params.senoidal.amplitud;

% v0 = perfil_params.polinomio7.vel.inicial;
% v1 = perfil_params.polinomio7.vel.final;
% 
% ac0 = perfil_params.polinomio7.acel.inicial;
% ac1 = perfil_params.polinomio7.acel.final;
% 
% j0 = perfil_params.polinomio7.jerk.inicial;
% j1 = perfil_params.polinomio7.jerk.inicial;

if perfil_params.senoidal.tiempo_inicio-1>0
    t0 = perfil_params.senoidal.tiempo_inicio-1;
else
    t0 = 0;
end
t1 = perfil_params.senoidal.tiempo_inicio;

% Coeficientes de un polinomio de 7mo grado
[qpol,vpol,apol,jpol] = pol7(t,q1,q0,t0,t1);

== matlab function Torque_controller_IFOC/Perfil torque de carga tau_L/If Action Subsystem4/Polinomio 7mo orden tau_L ==
  data: t input; perfil_params input; qpol output; vpol output; apol output; jpol output
function [qpol,vpol,apol,jpol] = fcn(t,perfil_params)

%Trayectoria de referencia

q0 = perfil_params.polinomio7.pos.inicial;
q1 = perfil_params.polinomio7.pos.final;

% v0 = perfil_params.polinomio7.vel.inicial;
% v1 = perfil_params.polinomio7.vel.final;
% 
% ac0 = perfil_params.polinomio7.acel.inicial;
% ac1 = perfil_params.polinomio7.acel.final;
% 
% j0 = perfil_params.polinomio7.jerk.inicial;
% j1 = perfil_params.polinomio7.jerk.inicial;

t0 = perfil_params.polinomio7.tiempo.inicial;
t1 = perfil_params.polinomio7.tiempo.final;

% Coeficientes de un polinomio de 7mo grado
[qpol,vpol,apol,jpol] = pol7(t,q0,q1,t0,t1);

== matlab function Torque_controller_IFOC/Perfil torque de carga tau_L/If Action Subsystem7/Trayectoria 15 segmentos ==
  data: t input size=1; q output size=1; perfil_params input
function q = fcn(t,perfil_params)

q0 = perfil_params.tr15segs.pos.inicial;
q1 = perfil_params.tr15segs.pos.final;

t0 = perfil_params.tr15segs.tiempo.inicial;

vel_path = perfil_params.tr15segs.vel_path;
acel_path = perfil_params.tr15segs.acel_path;
snap_path = perfil_params.tr15segs.snap_path;

dist = norm(q1-q0);
num_steps = 1000;




[interq,T] = pol15segs.bounded_tr(dist,num_steps,vel_path,acel_path,snap_path,0);

tstep = T/num_steps;
t1 = t0 + T;
t_tr = (t0:tstep:t1)';


[~,idt] = min(t_tr-t);
dire = (q1 - q0)/dist;
q = q0 + dire*interq(idt);

== matlab function Torque_controller_IFOC/Controlador IFOC/Perfil torque de carga tau_L/If Action Subsystem4/Polinomio 7mo orden tau_L ==
  data: t input; perfil_params input; qpol output; vpol output; apol output; jpol output
function [qpol,vpol,apol,jpol] = fcn(t,perfil_params)

%Trayectoria de referencia

q0 = perfil_params.polinomio7.pos.inicial;
q1 = perfil_params.polinomio7.pos.final;

% v0 = perfil_params.polinomio7.vel.inicial;
% v1 = perfil_params.polinomio7.vel.final;
% 
% ac0 = perfil_params.polinomio7.acel.inicial;
% ac1 = perfil_params.polinomio7.acel.final;
% 
% j0 = perfil_params.polinomio7.jerk.inicial;
% j1 = perfil_params.polinomio7.jerk.inicial;

t0 = perfil_params.polinomio7.tiempo.inicial;
t1 = perfil_params.polinomio7.tiempo.final;

% Coeficientes de un polinomio de 7mo grado
[qpol,vpol,apol,jpol] = pol7(t,q0,q1,t0,t1);

== matlab function Torque_controller_IFOC/Perfil torque de carga tau_L/If Action Subsystem6/Polinomio 7mo orden timeseries ==
  data: t input; qpol output; vpol output; apol output; jpol output
function [qpol,vpol,apol,jpol] = fcn(t)

q0 = 0;
q1 = 1;

t0 = 0.5;
t1 = 1;

%Trayectoria de referencia

% Coeficientes de un polinomio de 7mo grado
[qpol,vpol,apol,jpol] = pol7(t,q0,q1,t0,t1);

== matlab function Torque_controller_IFOC/Perfil torque de carga tau_L/If Action Subsystem/Senoidal tiempo de inicio ==
  data: t input; tr output; perfil_params input
function tr = fcn(t,perfil_params)

t1 = perfil_params.senoidal.tiempo_inicio;

if t < t1
    tr = 0;
else
    tr = t - t1;
end

== matlab function Torque_controller_IFOC/Perfil torque de carga tau_L/If Action Subsystem5/Tren de esca ==
  data: t input; q output; perfil_params input
function q = fcn(t,perfil_params)

q = Perfil_trayectoria.trEsca(t,perfil_params);

== matlab function Torque_controller_IFOC/Calculo de Potencia eléctrica/ab0 - ABC ==
  data: BPu input size=[2,1]; u output size=[3,1]
function u = fcn(BPu)

BPu = vertcat(BPu,0);

% Power invariant
BP = transforms.Clarke_transform(1);

u = BP^-1*BPu;

== matlab function Torque_controller_IFOC/Calculo de Potencia eléctrica/ab0 - ABC1 ==
  data: BPu input size=[2,1]; u output size=[3,1]
function u = fcn(BPu)

BPu = vertcat(BPu,0);

% Power invariant
BP = transforms.Clarke_transform(1);

u = BP^-1*BPu;

== matlab function Torque_controller_IFOC/Controlador IFOC/Perfil torque de carga tau_L/If Action Subsystem5/Tren de esca ==
  data: t input; q output; perfil_params input
function q = fcn(t,perfil_params)

q = Perfil_trayectoria.trEsca(t,perfil_params);

== matlab function Torque_controller_IFOC/Controlador IFOC/Perfil torque de carga tau_L/If Action Subsystem6/Polinomio 7mo orden timeseries ==
  data: t input; qpol output; vpol output; apol output; jpol output
function [qpol,vpol,apol,jpol] = fcn(t)

q0 = 0;
q1 = 1;

t0 = 0.5;
t1 = 1;

%Trayectoria de referencia

% Coeficientes de un polinomio de 7mo grado
[qpol,vpol,apol,jpol] = pol7(t,q0,q1,t0,t1);

== matlab function Torque_controller_IFOC/Controlador IFOC/Perfil torque de carga tau_L/If Action Subsystem7/Trayectoria 15 segmentos ==
  data: t input size=1; q output size=1; perfil_params input
function q = fcn(t,perfil_params)

q0 = perfil_params.tr15segs.pos.inicial;
q1 = perfil_params.tr15segs.pos.final;

t0 = perfil_params.tr15segs.tiempo.inicial;

vel_path = perfil_params.tr15segs.vel_path;
acel_path = perfil_params.tr15segs.acel_path;
snap_path = perfil_params.tr15segs.snap_path;

dist = norm(q1-q0);
num_steps = 1000;




[interq,T] = pol15segs.bounded_tr(dist,num_steps,vel_path,acel_path,snap_path,0);

tstep = T/num_steps;
t1 = t0 + T;
t_tr = (t0:tstep:t1)';


[~,idt] = min(t_tr-t);
dire = (q1 - q0)/dist;
q = q0 + dire*interq(idt);

== matlab function Torque_controller_IFOC/Controlador IFOC/Perfil torque de carga tau_L/If Action Subsystem/Polinomio 7mo orden sen ==
  data: t input; perfil_params input; qpol output; vpol output; apol output; jpol output
function [qpol,vpol,apol,jpol] = fcn(t,perfil_params)

%Trayectoria de referencia

q0 = 0;
q1 = perfil_params.senoidal.amplitud;

% v0 = perfil_params.polinomio7.vel.inicial;
% v1 = perfil_params.polinomio7.vel.final;
% 
% ac0 = perfil_params.polinomio7.acel.inicial;
% ac1 = perfil_params.polinomio7.acel.final;
% 
% j0 = perfil_params.polinomio7.jerk.inicial;
% j1 = perfil_params.polinomio7.jerk.inicial;

if perfil_params.senoidal.tiempo_inicio-1>0
    t0 = perfil_params.senoidal.tiempo_inicio-1;
else
    t0 = 0;
end
t1 = perfil_params.senoidal.tiempo_inicio;

% Coeficientes de un polinomio de 7mo grado
[qpol,vpol,apol,jpol] = pol7(t,q1,q0,t0,t1);

== matlab function Torque_controller_IFOC/Modelo MI (modelo ab)/ModeloMI ==
  data: MI_motor_params input; di_Sab output double size=[2 1]; dpsi_Rab output double size=[2 1]; dw_R output size=1; u_Sab input double size=[2 1]; i_Sab input double size=[2 1]; psi_Rab input double size=[2 1]; w_R input double size=1; tau_R output size=1; tau_L input
function [di_Sab,dpsi_Rab,dw_R,tau_R] = fcn(MI_motor_params,u_Sab,i_Sab,psi_Rab,w_R,tau_L)

[di_Sab,dpsi_Rab,dw_R,tau_R] = MI_model.MI_space_state(MI_motor_params,u_Sab,i_Sab,psi_Rab,w_R,tau_L);

== matlab function Torque_controller_IFOC/Controlador IFOC/Perfil torque de referencia tau_Rref/Polinomio 7mo orden tau_L ==
  data: t input; perfil_params input; qpol output; vpol output; apol output; jpol output
function [qpol,vpol,apol,jpol] = fcn(t,perfil_params)


% t,q0,q1,v0,v1,ac0,ac1,j0,j1,t0,t1)
%Trayectoria de referencia

q0 = perfil_params.polinomio7.pos.inicial;
q1 = perfil_params.polinomio7.pos.final;

v0 = perfil_params.polinomio7.vel.inicial;
v1 = perfil_params.polinomio7.vel.final;

ac0 = perfil_params.polinomio7.acel.inicial;
ac1 = perfil_params.polinomio7.acel.final;

j0 = perfil_params.polinomio7.jerk.inicial;
j1 = perfil_params.polinomio7.jerk.inicial;

t0 = perfil_params.polinomio7.tiempo.inicial;
t1 = perfil_params.polinomio7.tiempo.final;

% Coeficientes de un polinomio de 7mo grado

h = q1 - q0;
T = t1 - t0;

a = zeros(7+1,1);

a(1) = q0;
a(2) = v0;
a(3) = ac0/2;
a(4) = j0/6;
a(5) = (210*h-T*((30*ac0-15*ac1)*T+(4*j0+j1)*T^2+120*v0+90*v1))/(6*T^4);
a(6) = (-168*h-T*((20*ac0-14*ac1)*T+(2*j0+j1)*T^2+90*v0+78*v1))/(2*T^5);
a(7) = (420*h-T*((45*ac0-39*ac1)*T+(4*j0+3*j1)*T^2+216*v0+204*v1))/(6*T^6);
a(8) = (-120*h-T*((12*ac0-12*ac1)*T+(j0+j1)*T^2+60*v0+60*v1))/(6*T^7);

qa = flip(a')';
va = polyder(qa')';
aa = polyder(va')';
ja = polyder(aa')';


if t>=t0 && t<t1
    qpol = polyval(qa,t-t0);
    vpol = polyval(va,t-t0);
    apol = polyval(aa,t-t0);
    jpol = polyval(ja,t-t0);
elseif t>=t1
    qpol = polyval(qa,T);
    vpol = polyval(va,T);
    apol = polyval(aa,T);
    jpol = polyval(ja,T);
else
    qpol = 0;
    vpol = 0;
    apol = 0;
    jpol = 0;
end

== matlab function Torque_controller_IFOC/Controlador IFOC/Perfil torque de referencia tau_Rref/Polinomio 7mo orden timeseries ==
  data: t input; qpol output; vpol output; apol output; jpol output
function [qpol,vpol,apol,jpol] = fcn(t)


% t,q0,q1,v0,v1,ac0,ac1,j0,j1,t0,t1)
%Trayectoria de referencia

q0 = 0;
q1 = 1;

v0 = 0;
v1 = 0;

ac0 = 0;
ac1 = 0;

j0 = 0;
j1 = 0;

t0 = 0.5;
t1 = 1;

% Coeficientes de un polinomio de 7mo grado

h = q1 - q0;
T = t1 - t0;

a = zeros(7+1,1);

a(1) = q0;
a(2) = v0;
a(3) = ac0/2;
a(4) = j0/6;
a(5) = (210*h-T*((30*ac0-15*ac1)*T+(4*j0+j1)*T^2+120*v0+90*v1))/(6*T^4);
a(6) = (-168*h-T*((20*ac0-14*ac1)*T+(2*j0+j1)*T^2+90*v0+78*v1))/(2*T^5);
a(7) = (420*h-T*((45*ac0-39*ac1)*T+(4*j0+3*j1)*T^2+216*v0+204*v1))/(6*T^6);
a(8) = (-120*h-T*((12*ac0-12*ac1)*T+(j0+j1)*T^2+60*v0+60*v1))/(6*T^7);

qa = flip(a')';
va = polyder(qa')';
aa = polyder(va')';
ja = polyder(aa')';


if t>=t0 && t<t1
    qpol = polyval(qa,t-t0);
    vpol = polyval(va,t-t0);
    apol = polyval(aa,t-t0);
    jpol = polyval(ja,t-t0);
elseif t>=t1
    qpol = polyval(qa,T);
    vpol = polyval(va,T);
    apol = polyval(aa,T);
    jpol = polyval(ja,T);
else
    qpol = 0;
    vpol = 0;
    apol = 0;
    jpol = 0;
end

== matlab function Torque_controller_IFOC/Controlador IFOC/dq//ab ==
  data: i_sd input; i_sa output; i_sq input; rho input; i_sb output
function [i_sa,i_sb] = fcn(i_sd,i_sq,rho)

i_sa = cos(rho)*i_sd - sin(rho)*i_sq;
i_sb = sin(rho)*i_sd + cos(rho)*i_sq;

== matlab function Torque_controller_IFOC/Modelo MI (modelo ab)/ab//dq ==
  data: f input; f_d output; rho output
function [f_d,rho] = fcn(f)

[f_d,rho] = transforms.Polar_transform(f);

== matlab function Torque_controller_IFOC/Controlador IFOC/Perfil torque de carga tau_L/If Action Subsystem/Senoidal tiempo de inicio ==
  data: t input; tr output; perfil_params input
function tr = fcn(t,perfil_params)

t1 = perfil_params.senoidal.tiempo_inicio;

if t < t1
    tr = 0;
else
    tr = t - t1;
end
